simulink library "INT_ExtDem_SelectParameter"  (R2016b)
settings: Solver=VariableStepAuto  StartTime=0.0  StopTime=10.0  RelTol=1e-3
settings Model: Creator=xuxingpei  LastModifiedBy=xuxingpei

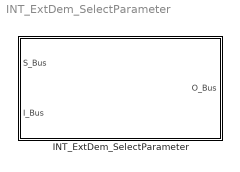
== system INT_ExtDem_SelectParameter ==
  INT_ExtDem_SelectParameter : Subsystem

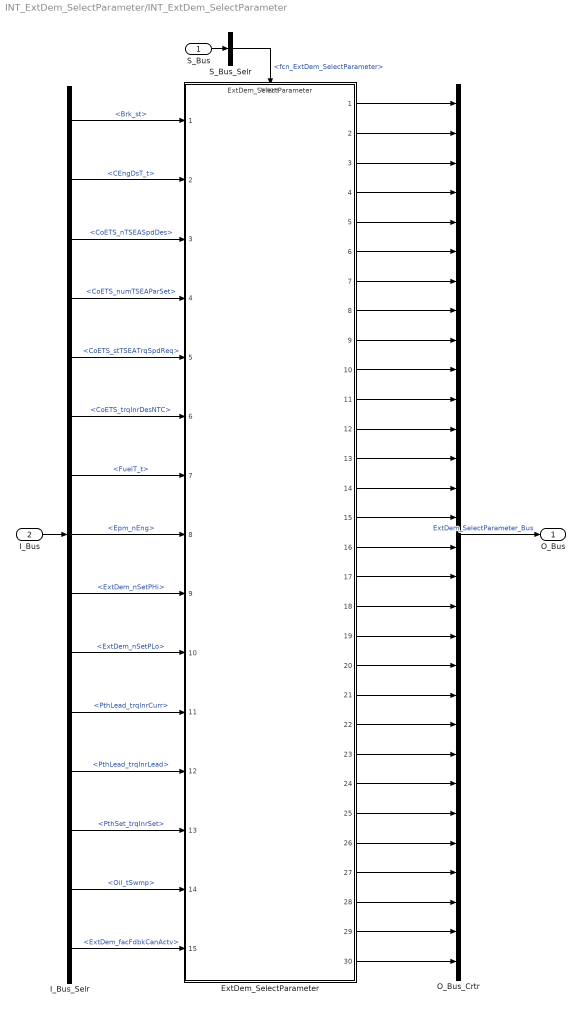
== system INT_ExtDem_SelectParameter/INT_ExtDem_SelectParameter ==
  S_Bus : Inport
  I_Bus : Inport  Port=2
  ExtDem_SelectParameter : ModelReference  ModelNameDialog=ExtDem_SelectParameter  SimulationMode=Normal  ModelReferenceVersion=1.210  TriggerPortName=function  TriggerPortTriggerType=function-call  TriggerPortStatesWhenEnabling=held
  I_Bus_Selr : BusSelector  OutputSignals=Brk_st,CEngDsT_t,CoETS_nTSEASpdDes,CoETS_numTSEAParSet,CoETS_stTSEATrqSpdReq,CoETS_trqInrDesNTC,FuelT_t,Epm_nEng,ExtDem_nSetPHi,ExtDem_nSetPLo,PthLead_trqInrCurr,PthLead_trqInrLead,PthSet_trqInrSet,Oil_tSwmp,ExtDem_facFdbkCanActv
  O_Bus_Crtr : BusCreator  Inputs=30
  S_Bus_Selr : BusSelector  OutputSignals=fcn_ExtDem_SelectParameter
  O_Bus : Outport
  wires:
  S_Bus_Selr/1 -> ExtDem_SelectParameter/Trigger  "<fcn_ExtDem_SelectParameter>"
  S_Bus/1 -> S_Bus_Selr/1
  I_Bus/1 -> I_Bus_Selr/1
  I_Bus_Selr/1 -> ExtDem_SelectParameter/1  "<Brk_st>"
  I_Bus_Selr/2 -> ExtDem_SelectParameter/2  "<CEngDsT_t>"
  I_Bus_Selr/3 -> ExtDem_SelectParameter/3  "<CoETS_nTSEASpdDes>"
  I_Bus_Selr/4 -> ExtDem_SelectParameter/4  "<CoETS_numTSEAParSet>"
  I_Bus_Selr/5 -> ExtDem_SelectParameter/5  "<CoETS_stTSEATrqSpdReq>"
  I_Bus_Selr/6 -> ExtDem_SelectParameter/6  "<CoETS_trqInrDesNTC>"
  I_Bus_Selr/7 -> ExtDem_SelectParameter/7  "<FuelT_t>"
  I_Bus_Selr/8 -> ExtDem_SelectParameter/8  "<Epm_nEng>"
  I_Bus_Selr/9 -> ExtDem_SelectParameter/9  "<ExtDem_nSetPHi>"
  I_Bus_Selr/10 -> ExtDem_SelectParameter/10  "<ExtDem_nSetPLo>"
  I_Bus_Selr/11 -> ExtDem_SelectParameter/11  "<PthLead_trqInrCurr>"
  I_Bus_Selr/12 -> ExtDem_SelectParameter/12  "<PthLead_trqInrLead>"
  I_Bus_Selr/13 -> ExtDem_SelectParameter/13  "<PthSet_trqInrSet>"
  I_Bus_Selr/14 -> ExtDem_SelectParameter/14  "<Oil_tSwmp>"
  I_Bus_Selr/15 -> ExtDem_SelectParameter/15  "<ExtDem_facFdbkCanActv>"
  O_Bus_Crtr/1 -> O_Bus/1  "ExtDem_SelectParameter_Bus"
  ExtDem_SelectParameter/1 -> O_Bus_Crtr/1
  ExtDem_SelectParameter/2 -> O_Bus_Crtr/2
  ExtDem_SelectParameter/3 -> O_Bus_Crtr/3
  ExtDem_SelectParameter/4 -> O_Bus_Crtr/4
  ExtDem_SelectParameter/5 -> O_Bus_Crtr/5
  ExtDem_SelectParameter/6 -> O_Bus_Crtr/6
  ExtDem_SelectParameter/7 -> O_Bus_Crtr/7
  ExtDem_SelectParameter/8 -> O_Bus_Crtr/8
  ExtDem_SelectParameter/9 -> O_Bus_Crtr/9
  ExtDem_SelectParameter/10 -> O_Bus_Crtr/10
  ExtDem_SelectParameter/11 -> O_Bus_Crtr/11
  ExtDem_SelectParameter/12 -> O_Bus_Crtr/12
  ExtDem_SelectParameter/13 -> O_Bus_Crtr/13
  ExtDem_SelectParameter/14 -> O_Bus_Crtr/14
  ExtDem_SelectParameter/15 -> O_Bus_Crtr/15
  ExtDem_SelectParameter/16 -> O_Bus_Crtr/16
  ExtDem_SelectParameter/17 -> O_Bus_Crtr/17
  ExtDem_SelectParameter/18 -> O_Bus_Crtr/18
  ExtDem_SelectParameter/19 -> O_Bus_Crtr/19
  ExtDem_SelectParameter/20 -> O_Bus_Crtr/20
  ExtDem_SelectParameter/21 -> O_Bus_Crtr/21
  ExtDem_SelectParameter/22 -> O_Bus_Crtr/22
  ExtDem_SelectParameter/23 -> O_Bus_Crtr/23
  ExtDem_SelectParameter/24 -> O_Bus_Crtr/24
  ExtDem_SelectParameter/25 -> O_Bus_Crtr/25
  ExtDem_SelectParameter/26 -> O_Bus_Crtr/26
  ExtDem_SelectParameter/27 -> O_Bus_Crtr/27
  ExtDem_SelectParameter/28 -> O_Bus_Crtr/28
  ExtDem_SelectParameter/29 -> O_Bus_Crtr/29
  ExtDem_SelectParameter/30 -> O_Bus_Crtr/30
